simulink model "emldemo_sort"  (R2015a)
settings: Solver=FixedStepDiscrete  StartTime=0.0  StopTime=10.0  FixedStep=10  RelTol=1e-3
CloseFcn:
  | rtwprivate ssgencode ModelCloseRequest my_sort
settings Model: CovSFcnEnable=off  Creator=The MathWorks, Inc.  LastModifiedBy=ktrinh
settings OptimizationCC: ExpressionDepthLimit=2147483647  InitFltsAndDblsToZero=on
settings DebuggingCC: SaveWithParameterizedLinksMsg=none  UnderspecifiedInitializationDetection=Classic  MergeDetectMultiDrivingBlocksExec=none  SignalResolutionControl=TryResolveAllWithWarning  SolverPrmCheckMsg=warning  MultiTaskDSMMsg=warning  MultiTaskCondExecSysMsg=none  FcnCallInpInsideContextMsg=EnableAllAsWarning  StateNameClashWarn=warning  StrictBusMsg=Warning
settings SFSimCC: SimCustomHeaderCode="#include \"c_sort.h\""  SimUserSources=c_sort.c  SimParseCustomCode=off
settings RTWCC: CustomInclude="#include \"c_sort.h\""  CustomSource=c_sort.c
settings GRTTargetCC: TargetFcnLib=ansi_tfl_tmw.mat  CombineOutputUpdateFcns=off  GRTInterface=on

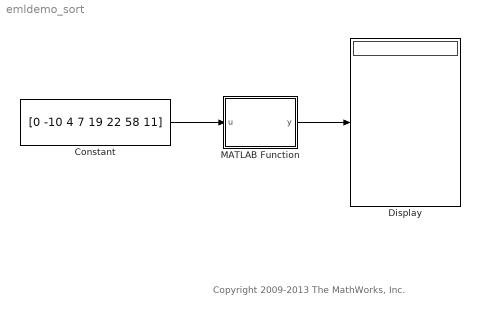
== system emldemo_sort ==
  note: Copyright 2009-2013 The MathWorks, Inc.
  Constant : Constant  Value=[0 -10 4 7 19 22 58 11]
  Display : Display
  MATLAB Function : MATLAB Function  TreatAsAtomicUnit=on
      settings: PermitHierarchicalResolution=ParametersOnly
  wires:
  Constant/1 -> MATLAB Function/1(u)
  MATLAB Function/1(y) -> Display/1

== matlab function emldemo_sort/MATLAB Function ==
  data: u input; y output
%#codegen
% The directive %#codegen is used to enable code generation messages in
% the MATLAB Code Analyzer.
function y = my_sort(u)

% Constrain 'y' to the same size and class as 'u'
y = u;

% Identify the MATLAB function 'disp' as an extrinsic function
coder.extrinsic('disp');

% Constrain the return type of function 'c_sort'
%   to a logical value
s = false;

% Call C function 'my_sort' with arguments:
%     coder.rref(y) - A read only reference to 'y'
%     coder.wref(y) - A write only reference to 'y'
%     numel(y)    - The number of elements of 'y' (or 'u')
s = coder.ceval('c_sort', coder.rref(y), coder.wref(y), int32(numel(y)));

if s % Already sorted
    disp('Already sorted.');
end
